simulink model "gm_sampleModel2081_2_sub_sub"  (R2023a)
settings: Solver=VariableStepAuto  StartTime=0.0  StopTime=10.0  RelTol=1e-3
libraries: hdlsllib x4, simulink x3
settings Model: Creator=user1  LastModifiedBy=user1
settings OptimizationCC: BlockReduction=off  ConditionallyExecuteInputs=off
settings DebuggingCC: InheritedTsInSrcMsg=none

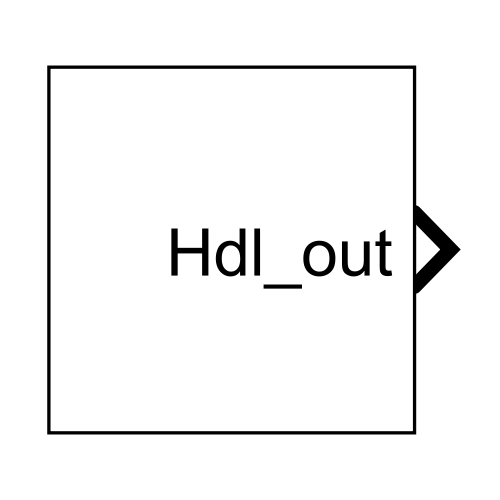
[thumbnail: Simulink's stored preview of the top-level diagram]
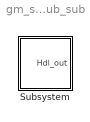
== system gm_sampleModel2081_2_sub_sub ==
  Subsystem : Subsystem

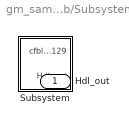
== system gm_sampleModel2081_2_sub_sub/Subsystem ==
  Subsystem : Subsystem
  Hdl_out : Outport  OutDataTypeStr=uint8

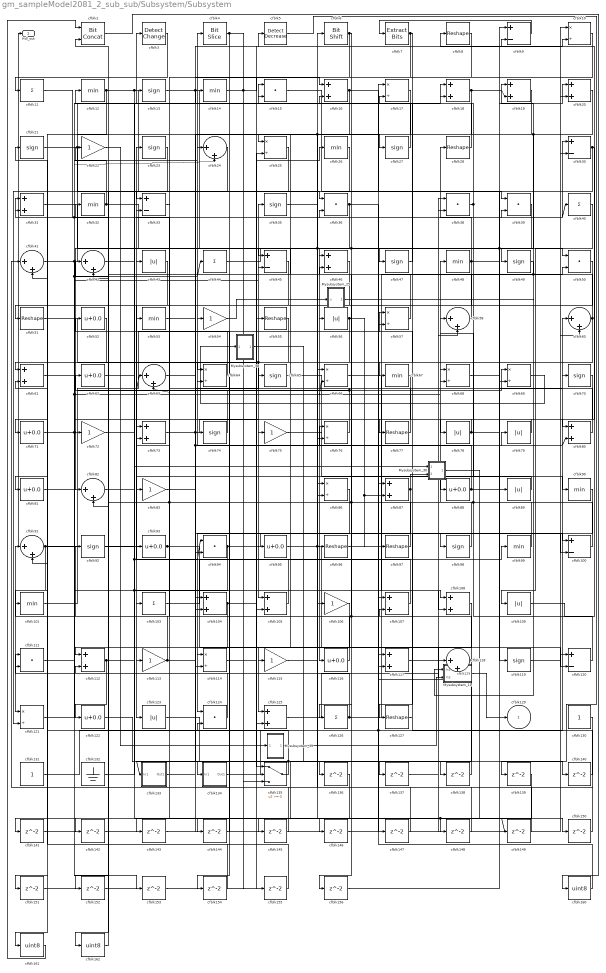
== system gm_sampleModel2081_2_sub_sub/Subsystem/Subsystem ==
  Mysubsystem_11 : Subsystem  TreatAsAtomicUnit=on  RTWFcnName=Mysubsystem_11
      settings: RTWFcnNameOpts=User specified  RTWFileNameOpts=Use function name
  Mysubsystem_25 : Subsystem  TreatAsAtomicUnit=on  RTWFcnName=Mysubsystem_25
      settings: RTWFcnNameOpts=User specified  RTWFileNameOpts=Use function name
  Mysubsystem_30 : Subsystem  TreatAsAtomicUnit=on  RTWFcnName=Mysubsystem_30
      settings: RTWFcnNameOpts=User specified  RTWFileNameOpts=Use function name
  Mysubsystem_38 : Subsystem  TreatAsAtomicUnit=on  RTWFcnName=Mysubsystem_38
      settings: RTWFcnNameOpts=User specified  RTWFileNameOpts=Use function name
  Mysubsystem_39 : Subsystem  TreatAsAtomicUnit=on  RTWFcnName=Mysubsystem_39
      settings: RTWFcnNameOpts=User specified  RTWFileNameOpts=Use function name
  cfblk{10,17,25,57,64,66,68..69,76,86,114,121} (12 alike) : Product  Inputs=*/  OutDataTypeStr=uint8  RndMeth=Zero  SaturateOnIntegerOverflow=on
  cfblk{9,30,33,45,100,120} (6 alike) : Sum  Inputs=+-  OutDataTypeStr=uint8
  cfblk{12,14,26,32,48,53,67,90,99,101} (10 alike) : MinMax  OutDataTypeStr=uint8
  cfblk{11,40,44,103,126} (5 alike) : Sum  Inputs=+  OutDataTypeStr=uint8
  cfblk{16,18..20,31,46,61,73,80,87,104..105,107..108,112,117,125} (17 alike) : Sum  OutDataTypeStr=uint8
  cfblk{22,54,72,75,83,106,113,115} (8 alike) : Gain  OutDataTypeStr=uint8
  cfblk{43,56,78..79,89,109,123} (7 alike) : Abs  OutDataTypeStr=uint8  SaturateOnIntegerOverflow=off
  cfblk{15,36,38..39,50,94,111,124} (8 alike) : DotProduct  OutDataTypeStr=uint8
  cfblk{52,62,71,81,88,93,95,116,122} (9 alike) : Bias  Bias=0.0  SaturateOnIntegerOverflow=off
  cfblk{24,41..42,58,60,63,82,91,118} (9 alike) : Sum  Inputs=|++  OutDataTypeStr=uint8
  cfblk{13,21,23,27,35,47,49,65,70,74,92,98,119} (13 alike) : Signum
  cfblk{8,28,51,55,77,96..97,127} (8 alike) : Reshape
  cfblk130 : Constant  OutDataTypeStr=uint8  SampleTime=-1
  cfblk131 : Constant  OutDataTypeStr=uint8  SampleTime=-1
  cfblk132 : Ground
  cfblk133 : Subsystem
      settings: LibrarySourceBlock=|
      | hdlsllib/Ports &
      | Subsystems/Subsystem
  cfblk134 : Subsystem
      settings: LibrarySourceBlock=|
      | hdlsllib/Ports &
      | Subsystems/Subsystem
  cfblk135 : Switch  OutDataTypeStr=uint8  SaturateOnIntegerOverflow=off  InputSameDT=off
  cfblk{136..156} (21 alike) : Delay  SampleTime=1
  cfblk160 : DataTypeConversion  OutDataTypeStr=uint8  SaturateOnIntegerOverflow=off  RndMeth=Floor
  cfblk161 : DataTypeConversion  OutDataTypeStr=uint8  SaturateOnIntegerOverflow=off  RndMeth=Floor
  cfblk162 : DataTypeConversion  OutDataTypeStr=uint8  SaturateOnIntegerOverflow=off  RndMeth=Floor
  cfblk2 : hdlsllib/Logic and Bit Operations/Bit Concat  numInputs=2
  cfblk3 : simulink/Logic and Bit Operations/Detect Change  vinit=0  OutDataTypeStr=uint8
      settings: LibrarySourceBlock=|
      | hdlsllib/Logic and Bit
      | Operations/Detect
      | Change
  cfblk4 : hdlsllib/Logic and Bit Operations/Bit Slice  lidx=7  ridx=0
  cfblk5 : simulink/Logic and Bit Operations/Detect Decrease  vinit=0.0  OutDataTypeStr=uint8
      settings: LibrarySourceBlock=|
      | hdlsllib/Logic and Bit
      | Operations/Detect
      | Decrease
  cfblk6 : hdlsllib/Logic and Bit Operations/Bit Shift  mode=Shift Left Logical  N=0
  cfblk7 : simulink/Logic and Bit Operations/Extract Bits  bitsToExtract=Upper half  numBits=8  bitIdxRange=[0 7]  outScalingMode=Preserve fixed-point scaling
      settings: LibrarySourceBlock=|
      | hdlsllib/Logic and Bit
      | Operations/Extract Bits
  cfblk129 : Outport  OutDataTypeStr=uint8  VectorParamsAs1DForOutWhenUnconnected=off
  Hdl_out : Outport  Port=2  OutDataTypeStr=uint8
  wires:
  cfblk101/1 -> cfblk69/1
  cfblk49/1 -> cfblk98/1
  cfblk40/1 -> cfblk109/1
  cfblk91/1 -> cfblk108/2, cfblk121/1
  cfblk28/1 -> cfblk12/1
  cfblk106/1 -> cfblk125/1
  cfblk116/1 -> cfblk92/1
  cfblk45/1 -> cfblk123/1
  cfblk58/1 -> cfblk82/1
  cfblk12/1 -> cfblk141/1, cfblk36/1, Mysubsystem_30/1(In1)
  cfblk113/1 -> cfblk65/1, cfblk91/1
  cfblk98/1 -> cfblk48/1
  cfblk44/1 -> cfblk50/1
  cfblk11/1 -> cfblk30/1
  cfblk107/1 -> cfblk23/1
  cfblk122/1 -> cfblk134/1(In1)
  cfblk133/1(Out1) -> cfblk80/2, cfblk36/2
  cfblk41/1 -> cfblk153/1, cfblk15/1
  cfblk36/1 -> cfblk140/1, cfblk116/1
  cfblk108/1 -> cfblk112/1
  cfblk35/1 -> cfblk149/1, cfblk148/1
  cfblk80/1 -> cfblk35/1
  cfblk17/1 -> cfblk95/1, cfblk86/2
  cfblk124/1 -> cfblk111/1
  cfblk74/1 -> cfblk62/1
  cfblk130/1 -> cfblk41/1
  cfblk117/1 -> cfblk118/1
  cfblk23/1 -> cfblk81/1
  cfblk57/1 -> cfblk43/1
  cfblk88/1 -> cfblk100/2, cfblk4/1
  cfblk56/1 -> cfblk97/1, cfblk87/2, cfblk71/1, cfblk105/1
  cfblk21/1 -> cfblk106/1, cfblk27/1
  cfblk109/1 -> cfblk8/1
  cfblk48/1 -> cfblk10/2, cfblk117/2, cfblk28/1
  cfblk13/1 -> cfblk16/2, cfblk16/1, cfblk47/1
  cfblk15/1 -> cfblk89/1
  cfblk134/1(Out1) -> cfblk60/1
  cfblk66/1 -> cfblk108/1
  cfblk115/1 -> cfblk99/1
  cfblk126/1 -> cfblk41/2, cfblk30/2
  cfblk8/1 -> cfblk103/1
  cfblk111/1 -> cfblk24/1, cfblk40/1
  cfblk67/1 -> cfblk115/1
  cfblk114/1 -> cfblk55/1
  cfblk3/1 -> cfblk11/1
  cfblk33/1 -> cfblk53/1
  cfblk135/1 -> cfblk21/1, cfblk133/1(In1)
  cfblk68/1 -> cfblk20/1
  cfblk100/1 -> cfblk63/2, cfblk42/1
  cfblk86/1 -> cfblk124/1
  cfblk87/1 -> cfblk156/1, Mysubsystem_30/2(In2)
  cfblk75/1 -> cfblk90/1
  cfblk132/1 -> cfblk68/2, cfblk94/1
  cfblk65/1 -> cfblk119/1
  cfblk47/1 -> cfblk17/2
  cfblk93/1 -> Hdl_out/1, cfblk120/2
  cfblk118/1 -> cfblk145/1, cfblk33/2, cfblk76/1
  cfblk120/1 -> cfblk68/1
  cfblk112/1 -> cfblk39/2, cfblk122/1
  cfblk31/1 -> cfblk46/1
  cfblk119/1 -> cfblk20/2
  cfblk6/1 -> cfblk33/1, cfblk56/1
  cfblk73/1 -> cfblk96/1, cfblk75/1
  cfblk79/1 -> cfblk78/1
  cfblk94/1 -> cfblk143/1, cfblk100/1
  cfblk125/1 -> cfblk79/1
  cfblk64/1 -> cfblk32/1
  cfblk61/1 -> cfblk24/2, cfblk44/1
  cfblk50/1 -> cfblk114/1
  cfblk14/1 -> cfblk135/3, cfblk9/2
  cfblk9/1 -> cfblk7/1
  cfblk60/1 -> cfblk101/1, cfblk31/2, cfblk19/1
  cfblk97/1 -> cfblk31/1, cfblk46/2
  cfblk96/1 -> cfblk50/2
  cfblk55/1 -> cfblk93/1
  cfblk92/1 -> cfblk15/2
  cfblk30/1 -> cfblk72/1, cfblk80/1
  cfblk18/1 -> cfblk25/1, cfblk19/2
  cfblk46/1 -> cfblk73/1
  cfblk4/1 -> cfblk155/1, cfblk154/1
  cfblk95/1 -> cfblk118/2, cfblk6/1
  cfblk25/1 -> cfblk64/1
  cfblk24/1 -> cfblk51/1
  cfblk82/1 -> cfblk136/1, cfblk104/2
  cfblk27/1 -> cfblk3/1
  cfblk71/1 -> cfblk45/2, cfblk57/1
  cfblk51/1 -> cfblk135/1
  cfblk83/1 -> cfblk5/1
  cfblk131/1 -> cfblk10/1, cfblk87/1
  cfblk39/1 -> cfblk69/2, cfblk42/2, cfblk126/1
  cfblk16/1 -> cfblk114/2, cfblk39/1
  cfblk76/1 -> cfblk54/1, cfblk63/1
  cfblk105/1 -> cfblk74/1
  cfblk62/1 -> cfblk18/1
  cfblk78/1 -> cfblk70/1, cfblk77/1
  cfblk104/1 -> cfblk26/1, cfblk113/1
  cfblk81/1 -> cfblk14/1
  cfblk121/1 -> cfblk66/2, cfblk13/1
  cfblk7/1 -> cfblk105/2, cfblk67/1
  cfblk90/1 -> cfblk127/1
  cfblk38/1 -> cfblk88/1, cfblk18/2
  cfblk20/1 -> cfblk45/1, cfblk49/1
  cfblk32/1 -> cfblk22/1, cfblk117/1, cfblk66/1
  cfblk127/1 -> cfblk57/2
  cfblk26/1 -> cfblk121/2
  cfblk77/1 -> cfblk52/1
  cfblk53/1 -> cfblk94/2
  cfblk103/1 -> cfblk38/2
  cfblk43/1 -> cfblk61/1
  cfblk99/1 -> cfblk73/2, cfblk58/1
  cfblk19/1 -> cfblk76/2
  cfblk89/1 -> cfblk83/1
  cfblk63/1 -> cfblk137/1
  cfblk137/1 -> cfblk38/1
  cfblk138/1 -> cfblk17/1
  cfblk5/1 -> cfblk139/1
  cfblk140/1 -> cfblk107/2
  cfblk141/1 -> cfblk58/2
  cfblk142/1 -> cfblk104/1
  cfblk143/1 -> cfblk60/2
  cfblk42/1 -> cfblk144/1
  cfblk144/1 -> cfblk64/2
  cfblk145/1 -> cfblk61/2
  cfblk10/1 -> cfblk146/1
  cfblk146/1 -> cfblk120/1
  cfblk123/1 -> cfblk147/1
  cfblk147/1 -> cfblk124/2
  cfblk148/1 -> cfblk86/1
  cfblk149/1 -> cfblk112/2
  cfblk72/1 -> cfblk150/1
  cfblk150/1 -> cfblk135/2
  cfblk52/1 -> cfblk151/1
  cfblk151/1 -> cfblk125/2
  cfblk70/1 -> cfblk152/1
  cfblk152/1 -> cfblk82/2
  cfblk153/1 -> cfblk25/2
  cfblk154/1 -> cfblk91/2
  cfblk155/1 -> cfblk111/2
  cfblk156/1 -> cfblk9/1
  cfblk2/1 -> cfblk160/1
  cfblk160/1 -> cfblk107/1
  cfblk139/1 -> cfblk161/1
  cfblk161/1 -> cfblk2/1
  cfblk136/1 -> cfblk162/1
  cfblk162/1 -> cfblk2/2
  Mysubsystem_11/1(cfblk129) -> cfblk129/1
  cfblk54/1 -> Mysubsystem_25/1(u)
  Mysubsystem_25/1(Out1) -> Mysubsystem_11/1(In1)
  Mysubsystem_30/1(Out1) -> cfblk142/1
  cfblk69/1 -> Mysubsystem_38/1(In1)
  Mysubsystem_38/1(Out1) -> cfblk138/1
  cfblk22/1 -> Mysubsystem_39/1(In1)
  Mysubsystem_39/1(Out1) -> Mysubsystem_11/2(In2)

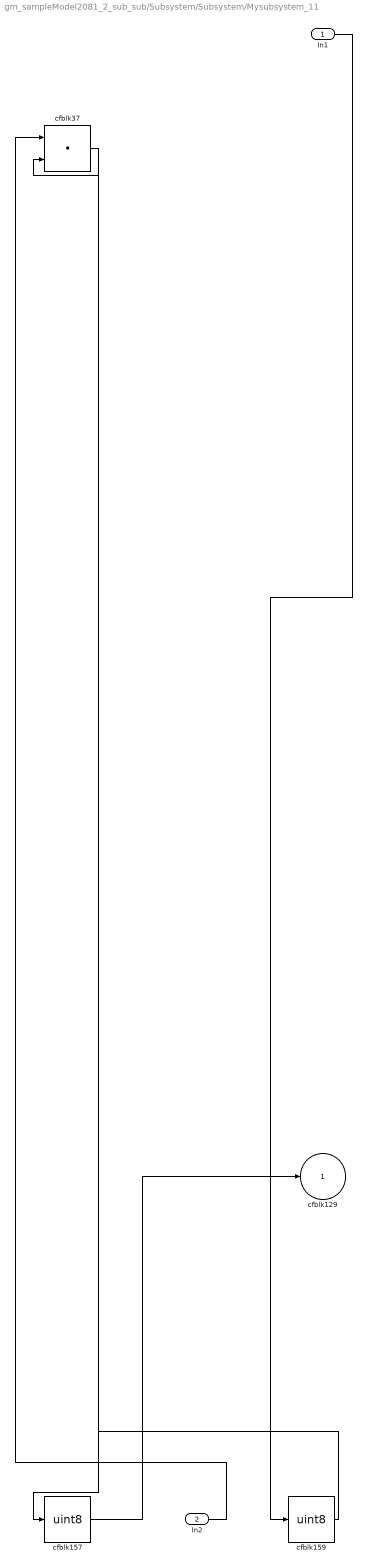
== system gm_sampleModel2081_2_sub_sub/Subsystem/Subsystem/Mysubsystem_11 ==
  In1 : Inport
  In2 : Inport  Port=2
  cfblk157 : DataTypeConversion  OutDataTypeStr=uint8  SaturateOnIntegerOverflow=off  RndMeth=Floor
  cfblk159 : DataTypeConversion  OutDataTypeStr=uint8  SaturateOnIntegerOverflow=off  RndMeth=Floor
  cfblk37 : DotProduct  OutDataTypeStr=Inherit: Inherit via internal rule
  cfblk129 : Outport  VectorParamsAs1DForOutWhenUnconnected=off
  wires:
  cfblk157/1 -> cfblk129/1
  cfblk37/1 -> cfblk157/1
  In2/1 -> cfblk37/1
  cfblk159/1 -> cfblk37/2
  In1/1 -> cfblk159/1

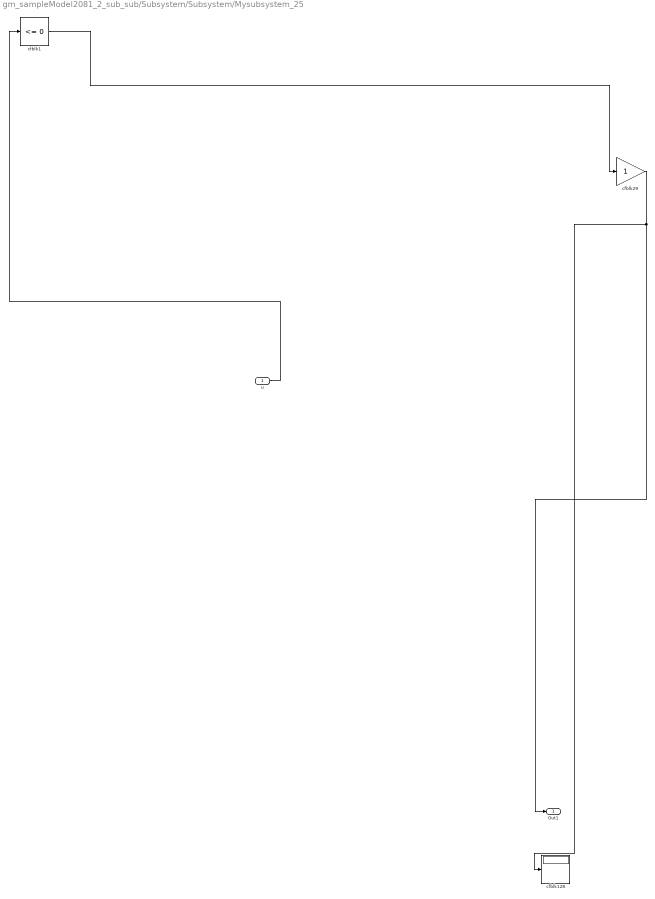
== system gm_sampleModel2081_2_sub_sub/Subsystem/Subsystem/Mysubsystem_25 ==
  u : Inport
  cfblk1 : hdlsllib/Logic and Bit Operations/Compare To Zero  relop=<=  OutDataTypeStr=boolean
  cfblk128 : Display
  cfblk29 : Gain
  Out1 : Outport
  wires:
  u/1 -> cfblk1/1
  cfblk1/1 -> cfblk29/1
  cfblk29/1 -> cfblk128/1, Out1/1

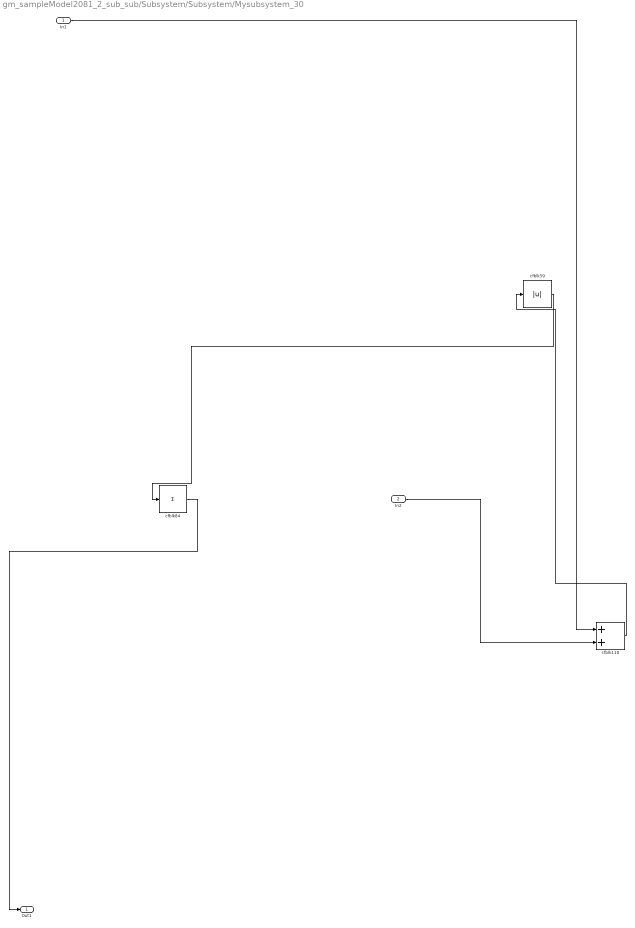
== system gm_sampleModel2081_2_sub_sub/Subsystem/Subsystem/Mysubsystem_30 ==
  In1 : Inport
  In2 : Inport  Port=2
  cfblk110 : Sum
  cfblk59 : Abs  SaturateOnIntegerOverflow=off
  cfblk84 : Sum  Inputs=+
  Out1 : Outport
  wires:
  In1/1 -> cfblk110/1
  In2/1 -> cfblk110/2
  cfblk110/1 -> cfblk59/1
  cfblk84/1 -> Out1/1
  cfblk59/1 -> cfblk84/1

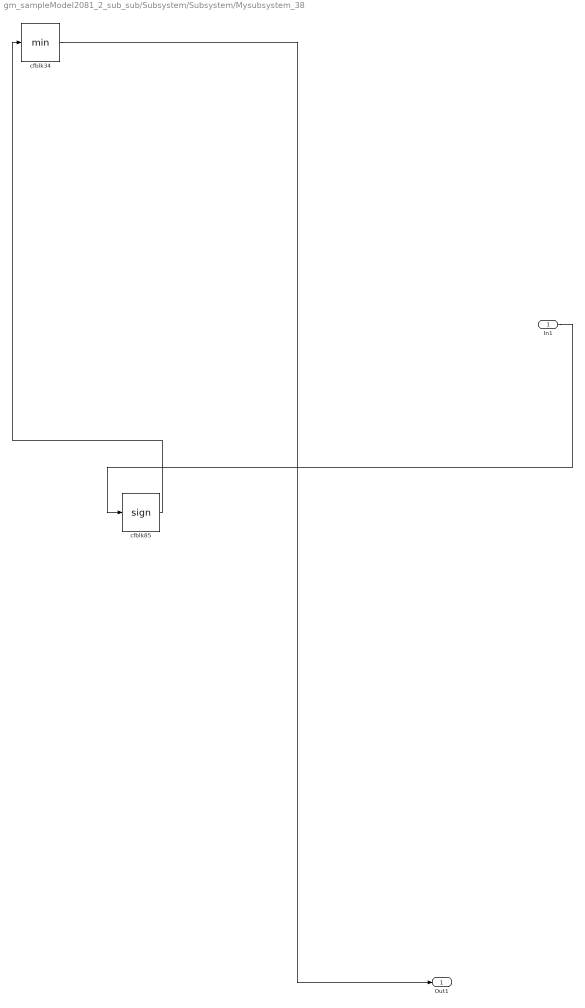
== system gm_sampleModel2081_2_sub_sub/Subsystem/Subsystem/Mysubsystem_38 ==
  In1 : Inport
  cfblk34 : MinMax
  cfblk85 : Signum
  Out1 : Outport
  wires:
  In1/1 -> cfblk85/1
  cfblk85/1 -> cfblk34/1
  cfblk34/1 -> Out1/1

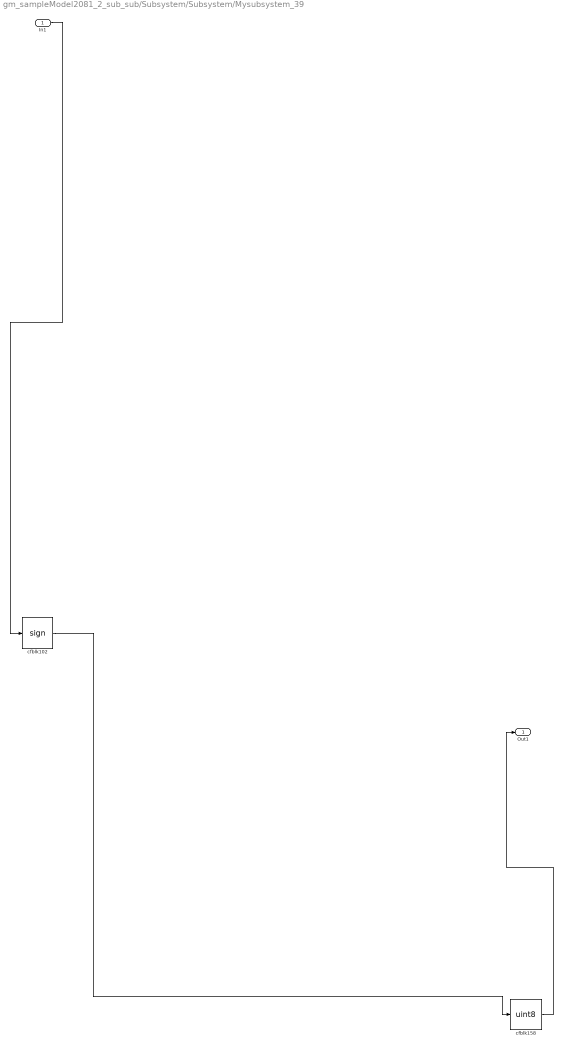
== system gm_sampleModel2081_2_sub_sub/Subsystem/Subsystem/Mysubsystem_39 ==
  In1 : Inport
  cfblk102 : Signum
  cfblk158 : DataTypeConversion  OutDataTypeStr=uint8  SaturateOnIntegerOverflow=off  RndMeth=Floor
  Out1 : Outport
  wires:
  In1/1 -> cfblk102/1
  cfblk158/1 -> Out1/1
  cfblk102/1 -> cfblk158/1

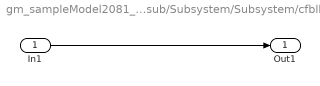
== system gm_sampleModel2081_2_sub_sub/Subsystem/Subsystem/cfblk133 ==
  In1 : Inport
  Out1 : Outport
  wires:
  In1/1 -> Out1/1

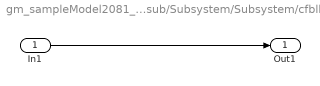
== system gm_sampleModel2081_2_sub_sub/Subsystem/Subsystem/cfblk134 ==
  In1 : Inport
  Out1 : Outport
  wires:
  In1/1 -> Out1/1
